simulink model "ECE664_Project_model_exp2"  (R2018b)
settings: Solver=VariableStepAuto  StartTime=0.0  StopTime=0.1  MaxStep=1E-6  RelTol=1E-5
values from neighbouring files (symbols this model uses):
  Ac = [0 1; -(w^2)-kf -2*Xi*w]    [Deadbeat.m]
  Bc = [0; gss*ku]    [Deadbeat.m]
  K = acker(Ad, Bd, poles)    [Deadbeat.m]
  L = K'    [Deadbeat.m]    (also in Deadbeat2.m = Q*[b0-a0; b1-a1])
  Ts = 0.0001    [Deadbeat.m]    (also in Deadbeat2.m)
undefined symbols (not defined in the file or in its folder): C, x0
settings Model: Creator=Biao Cheng  LastModifiedBy=ohara

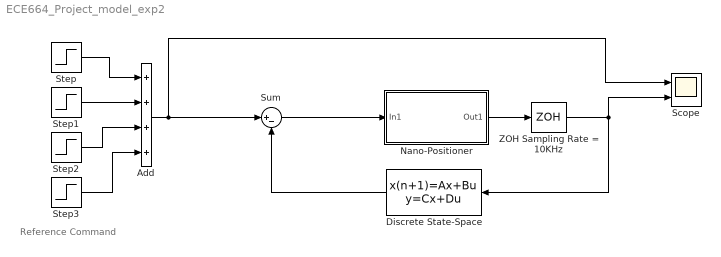
== system ECE664_Project_model_exp2 ==
  note: Reference Command
  Add : Sum  Inputs=++++
  Discrete State-Space : DiscreteStateSpace  A=Ac+Bc*K-L*C  B=L  C=K  D=0  InitialCondition=x0  SampleTime=Ts
  Nano-Positioner : Subsystem
  Scope : Scope  NumInputPorts=2
  Step : Step  Time=5E-3  SampleTime=0
  Step1 : Step  Time=15E-3  SampleTime=0
  Step2 : Step  Time=25E-3  After=-1  SampleTime=0
  Step3 : Step  Time=35E-3  After=-1  SampleTime=0
  Sum : Sum  Inputs=|+-
  ZOH Sampling Rate = 10KHz : ZeroOrderHold  SampleTime=1E-5
  wires:
  Step/1 -> Add/1
  Step1/1 -> Add/2
  Step2/1 -> Add/3
  Step3/1 -> Add/4
  Add/1 -> Sum/1, Scope/1
  Nano-Positioner/1(Out1) -> ZOH Sampling Rate = 10KHz/1
  Sum/1 -> Nano-Positioner/1(In1)
  Discrete State-Space/1 -> Sum/2
  ZOH Sampling Rate = 10KHz/1 -> Discrete State-Space/1, Scope/2

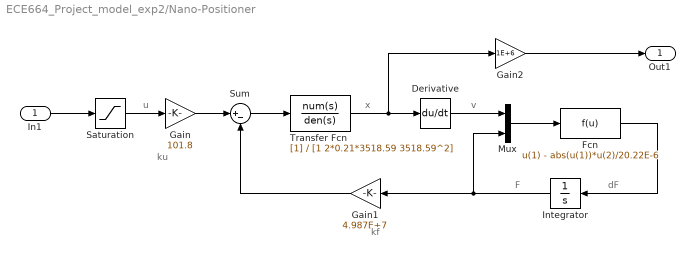
== system ECE664_Project_model_exp2/Nano-Positioner ==
  note: dF
  note: F
  note: v
  note: x
  note: kf
  note: u
  note: ku
  In1 : Inport
  Derivative : Derivative
  Fcn : Fcn  Expr=u(1) - abs(u(1))*u(2)/20.22E-6
  Gain : Gain  Gain=101.8
  Gain1 : Gain  Gain=4.987E+7
  Gain2 : Gain  Gain=1E+6
  Integrator : Integrator
  Mux : Mux  Inputs=2
  Saturation : Saturate  UpperLimit=4  LowerLimit=-4
  Sum : Sum  Inputs=|+-
  Transfer Fcn : TransferFcn  Denominator=[1 2*0.21*3518.59 3518.59^2]
  Out1 : Outport
  wires:
  Gain1/1 -> Sum/2
  Mux/1 -> Fcn/1
  Integrator/1 -> Mux/2, Gain1/1
  In1/1 -> Saturation/1
  Derivative/1 -> Mux/1
  Fcn/1 -> Integrator/1
  Sum/1 -> Transfer Fcn/1
  Saturation/1 -> Gain/1
  Gain/1 -> Sum/1
  Transfer Fcn/1 -> Gain2/1, Derivative/1
  Gain2/1 -> Out1/1
